simulink model "Testdistancia"  (R2023b)
settings: Solver=VariableStepAuto  StartTime=0.0  StopTime=10.0  RelTol=1e-3
settings Model: Creator=USUARIO  LastModifiedBy=USUARIO

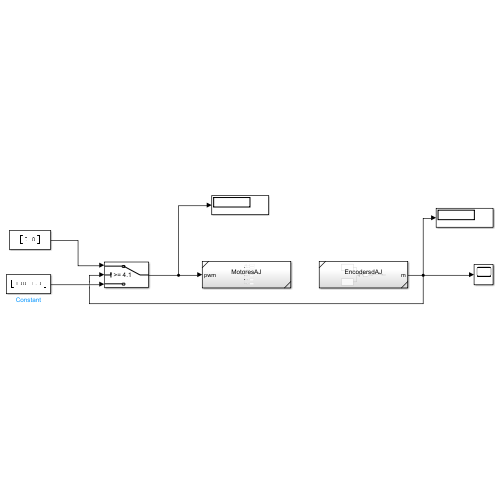
[thumbnail: Simulink's stored preview of the top-level diagram]
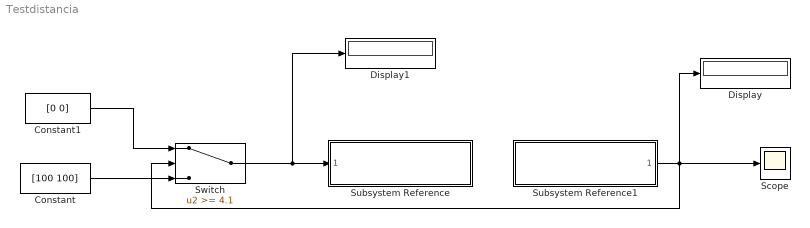
== system Testdistancia ==
  Constant : Constant  Value=[100 100]
  Constant1 : Constant  Value=[0 0]
  Display : Display
  Display1 : Display
  Scope : Scope
  Subsystem Reference : Subsystem  ReferencedSubsystem=MotoresAJ
  Subsystem Reference1 : Subsystem  ReferencedSubsystem=EncodersdAJ
  Switch : Switch  Threshold=4.1  SaturateOnIntegerOverflow=off  InputSameDT=off
  wires:
  Switch/1 -> Display1/1, Subsystem Reference/1
  Subsystem Reference1/1 -> Scope/1, Display/1, Switch/2
  Constant1/1 -> Switch/1
  Constant/1 -> Switch/3
